simulink model "velexample5classv2023v2"  (R2021b)
settings: Solver=ode3  StartTime=0.0  StopTime=10  FixedStep=ts  RelTol=1e-3  EnableMultiTasking=on
undefined symbols (not defined in the file): ts
libraries: arduinolib x3, simulink x1, arduinosensorlib x1, dspstat3 x1
settings Model: ExtModeTrigDuration=2  Creator=tsuga  LastModifiedBy=karteek
settings SolverCC: AutoInsertRateTranBlk=on
settings DataIOCC: SaveOutput=off  DSMLogging=off  SaveTime=off  ReturnWorkspaceOutputs=off
settings OptimizationCC: DefaultParameterBehavior=Inlined  StrengthReduction=on  PassReuseOutputArgsAs=Individual arguments  ZeroExternalMemoryAtStartup=off  ZeroInternalMemoryAtStartup=off  MaxStackSize=64  OptimizeBlockOrder=speed  OptimizationPriority=Speed  OptimizationCustomize=off  MultiThreadedLoops=on  EfficientTunableParamExpr=on
settings DebuggingCC: ParameterTunabilityLossMsg=error
settings HardwareCC: ProdBitPerInt=16  ProdBitPerPointer=16  ProdBitPerSizeT=16  ProdBitPerPtrDiffT=16  ProdLargestAtomicFloat=None  ProdWordSize=8  ProdHWDeviceType=Atmel->AVR
settings SFSimCC: MATLABDynamicMemAlloc=off
settings RTWCC: Description=Embedded Coder  SystemTargetFile=ert.tlc  HardwareBoard=Arduino Leonardo  TemplateMakefile=ert_default_tmf  Toolchain=Arduino AVR  BuildConfiguration=Faster Runs
settings CodeAppCC: ForceParamTrailComments=on  IgnoreCustomStorageClasses=off  OperatorAnnotations=on  SimulinkDataObjDesc=on  SFDataObjDesc=on  InsertBlockDesc=on
settings ERTTargetCC: SupportContinuousTime=on  SupportVariableSizeSignals=on  ExtModeTransport=5  ExtModeStaticAllocSize=250  ExtModeMexFile=ext_serial_win32_comm_leonardo

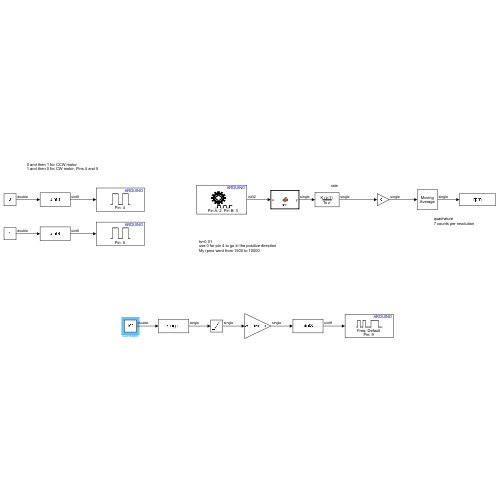
[thumbnail: Simulink's stored preview of the top-level diagram]
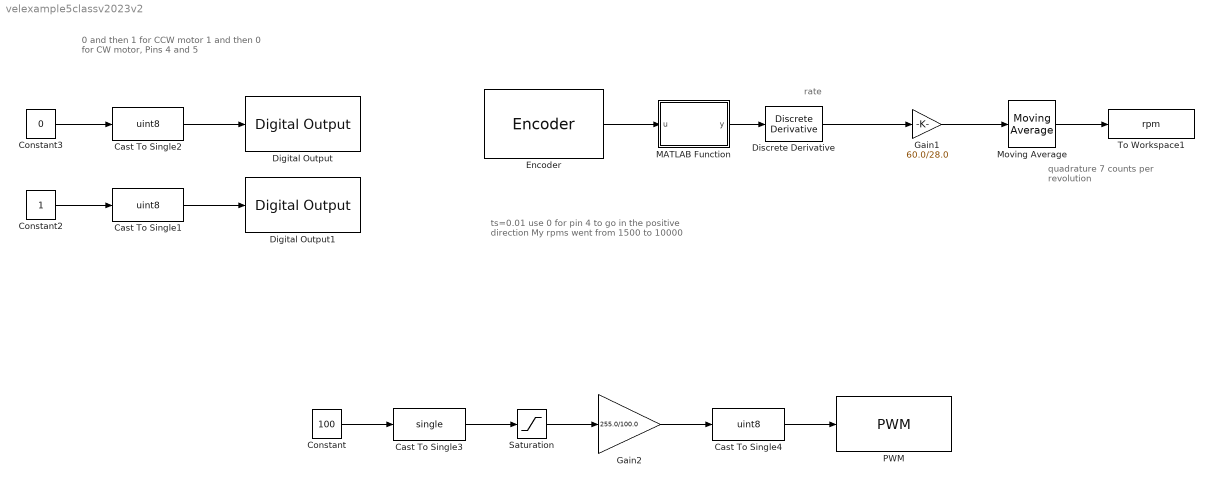
== system velexample5classv2023v2 ==
  note: rate
  note: quadrature
      | 7 counts per revolution
  note: ts=0.01
      | use 0 for pin 4 to go in the positive direction
      | My rpms went from 1500 to 10000
  note: 0 and then 1 for CCW motor
      | 1 and then 0 for CW motor, Pins 4 and 5
  Cast To Single1 : DataTypeConversion  OutDataTypeStr=uint8
  Cast To Single2 : DataTypeConversion  OutDataTypeStr=uint8
  Cast To Single3 : DataTypeConversion  OutDataTypeStr=single
  Cast To Single4 : DataTypeConversion  OutDataTypeStr=uint8
  Constant : Constant  Value=100  SampleTime=ts
  Constant2 : Constant  SampleTime=ts
  Constant3 : Constant  Value=0  SampleTime=ts
  Digital Output : arduinolib/Digital Output  pinNumber=4  Direction=output  blockPlatform=arduino
  Digital Output1 : arduinolib/Digital Output  pinNumber=5  Direction=output  blockPlatform=arduino
  Discrete Derivative : simulink/Discrete/Discrete Derivative  gainval=1.0  ICPrevScaledInput=0.0  OutMin=[]  OutMax=[]  OutDataType=fixdt(1, 16)  OutScaling=2^-10  DoSatur=off
  Encoder : arduinosensorlib/Encoder  InputA=2  InputB=3  Mode=No reset  SampleTime=ts
      settings: SourceProductBaseCode=ARDUINO
  Gain1 : Gain  Gain=60.0/28.0
  Gain2 : Gain  Gain=255.0/100.0
  MATLAB Function : MATLAB Function  TreatAsAtomicUnit=on
  Moving Average : dspstat3/Moving Average  Method=Sliding window  ForgettingFactorPort=off  SpecifyWindowLength=on  WindowLength=4  ForgettingFactor=0.9  SimulateUsing=Code generation
  PWM : arduinolib/PWM  pinNumber=9  frequencyType=Default  desiredFrequency=490.2  achievableFrequency=490.2
  Saturation : Saturate  UpperLimit=100.0  LowerLimit=0.0
  To Workspace1 : ToWorkspace  VariableName=rpm  SampleTime=ts
      settings: Save2DSignal=2-D array (concatenate along first dimension)
  wires:
  Cast To Single3/1 -> Saturation/1
  Saturation/1 -> Gain2/1
  Gain2/1 -> Cast To Single4/1
  Cast To Single4/1 -> PWM/1
  Constant2/1 -> Cast To Single1/1
  Cast To Single1/1 -> Digital Output1/1
  Cast To Single2/1 -> Digital Output/1
  Constant3/1 -> Cast To Single2/1
  MATLAB Function/1(y) -> Discrete Derivative/1
  Encoder/1 -> MATLAB Function/1(u)
  Discrete Derivative/1 -> Gain1/1
  Gain1/1 -> Moving Average/1
  Moving Average/1 -> To Workspace1/1
  Constant/1 -> Cast To Single3/1

== matlab function velexample5classv2023v2/MATLAB Function ==
  data: u input; y output
function y = fcn(u)
%#codegen

% xx = typecast(u,'single');
% y=xx(1);

y=single(u);  % this method worked
